simulink model "dsm_l2_sim"  (R2024b)
settings: Solver=FixedStepDiscrete  StartTime=0.0  StopTime=1024  RelTol=1e-3  AbsTol=1e-6
values from neighbouring files (symbols this model uses):
  Ts = 1/fs    (= 4.54545454545e-06)    [dsm_l2_sim.m]    (also in dsm_l2_sim_code.m)
undefined symbols (not defined in the file or in its folder): a, b, c
settings Model: Creator=mimeiners  LastModifiedBy=nicki
settings SolverCC: AutoScaleAbsTol=off  AlgebraicLoopSolver=TrustRegion
settings DataIOCC: SaveFormat=Array  SignalLoggingSaveFormat=ModelDataLogs  SignalLogging=off  DSMLogging=off  SaveTime=off  ReturnWorkspaceOutputs=off  SignalLoggingName=sigsOut
settings OptimizationCC: BooleanDataType=off  ReuseModelBlockBuffer=off
settings DebuggingCC: SaveWithParameterizedLinksMsg=none  UnderspecifiedInitializationDetection=Classic  MergeDetectMultiDrivingBlocksExec=none  SignalResolutionControl=TryResolveAllWithWarning  MultiTaskDSMMsg=warning  MultiTaskCondExecSysMsg=none  UnconnectedInputMsg=warning  UnconnectedOutputMsg=warning  UnconnectedLineMsg=warning  ArithmeticOperatorsInVariantConditions=warning
settings HardwareCC: ProdBitPerPointer=32  ProdBitPerSizeT=32  ProdBitPerPtrDiffT=32  ProdLargestAtomicFloat=None  ProdIntDivRoundTo=Undefined  ProdEndianess=Unspecified  ProdWordSize=32  ProdHWDeviceType=32-bit Generic  TargetUnknown=on
settings ModelReferenceCC: EnableRefExpFcnMdlSchedulingChecks=on  PropagateSignalLabelsOutOfModel=off
settings SFSimCC: SimUseLocalCustomCode=off  CustomCodeUndefinedFunction=UseInterfaceOnly
settings RTWCC: TemplateMakefile=grt_vc.tmf  RTWUseLocalCustomCode=off  GPUComputeCapability=3.5
settings GRTTargetCC: TargetLangStandard=C89/C90 (ANSI)  CombineOutputUpdateFcns=off  GRTInterface=on
settings ConfigComp: CovMetricSettings=dw  CovSaveCumulativeToWorkspaceVar=on  CovSaveSingleToWorkspaceVar=on  CovExternalEMLEnable=off

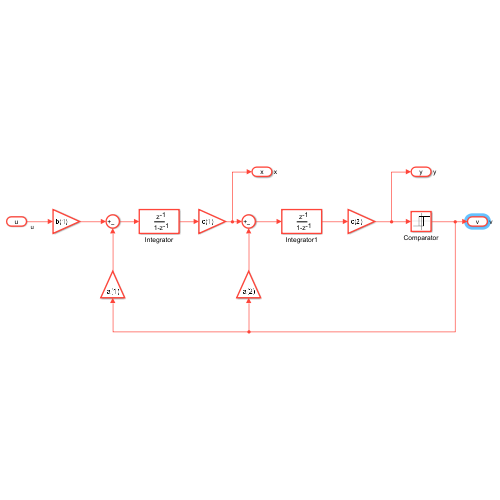
[thumbnail: Simulink's stored preview of the top-level diagram]
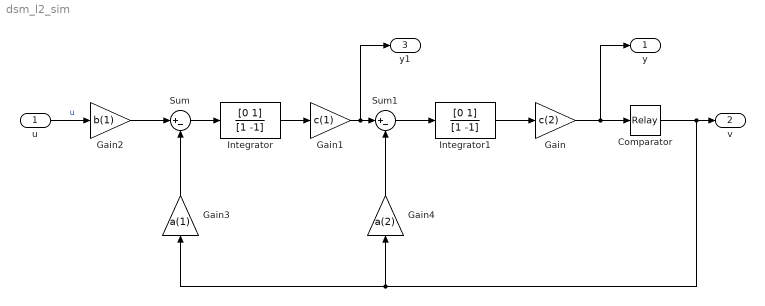
== system dsm_l2_sim ==
  u : Inport
  Comparator : Relay  OffOutputValue=-1
  Gain : Gain  Gain=c(2)
  Gain1 : Gain  Gain=c(1)
  Gain2 : Gain  Gain=b(1)
  Gain3 : Gain  Gain=a(1)
  Gain4 : Gain  Gain=a(2)
  Integrator : DiscreteFilter  Numerator=[0 1]  Denominator=[1 -1]  SampleTime=Ts
  Integrator1 : DiscreteFilter  Numerator=[0 1]  Denominator=[1 -1]  SampleTime=Ts
  Sum : Sum  Inputs=|+-  InputSameDT=on  SaturateOnIntegerOverflow=on  OutDataTypeStr=Inherit: Same as first input
  Sum1 : Sum  Inputs=|+-  InputSameDT=on  SaturateOnIntegerOverflow=on  OutDataTypeStr=Inherit: Same as first input
  y : Outport  SignalName=y  VectorParamsAs1DForOutWhenUnconnected=off
  v : Outport  Port=2  SignalName=v  VectorParamsAs1DForOutWhenUnconnected=off
  y1 : Outport  Port=3  SignalName=x  VectorParamsAs1DForOutWhenUnconnected=off
  wires:
  Sum/1 -> Integrator/1
  Gain2/1 -> Sum/1
  Integrator/1 -> Gain1/1
  Sum1/1 -> Integrator1/1
  Integrator1/1 -> Gain/1
  Gain/1 -> y/1, Comparator/1
  Gain3/1 -> Sum/2
  Gain4/1 -> Sum1/2
  Comparator/1 -> Gain4/1, Gain3/1, v/1
  u/1 -> Gain2/1  "u"
  Gain1/1 -> y1/1, Sum1/1
